simulink model "verify_clq2pressuredropcoeff_mdl"  (R2016b)
settings: Solver=VariableStepDiscrete  StartTime=0.0  StopTime=10.0  MaxStep=0.1  RelTol=1e-3  EnableMultiTasking=on
libraries: carnot x3, simulink x1
settings Model: Creator=drhf  LastModifiedBy=drhf
settings DataIOCC: LimitDataPoints=on  SaveFormat=Array
settings OptimizationCC: ExpressionDepthLimit=2147483647  LifeSpan=inf
settings DebuggingCC: UnderspecifiedInitializationDetection=Classic  MergeDetectMultiDrivingBlocksExec=none  SolverPrmCheckMsg=warning  StateNameClashWarn=warning  SFUnexpectedBacktrackingDiag=warning  SFNoUnconditionalDefaultTransitionDiag=warning  SFExecutionAtInitializationDiag=none
settings HardwareCC: ProdBitPerPointer=32  ProdBitPerSizeT=32  ProdBitPerPtrDiffT=32  ProdLargestAtomicFloat=None  ProdIntDivRoundTo=Undefined  ProdEndianess=Unspecified  ProdWordSize=32  ProdHWDeviceType=32-bit Generic
settings ModelReferenceCC: PropagateSignalLabelsOutOfModel=off
settings GRTTargetCC: TargetLangStandard=C89/C90 (ANSI)  GeneratePreprocessorConditionals=Disable all  CombineOutputUpdateFcns=off  GRTInterface=on
settings ConfigComp: CovMetricSettings=dw  CovHtmlReporting=on  CovSaveCumulativeToWorkspaceVar=on  CovSaveSingleToWorkspaceVar=on  CovExternalEMLEnable=off

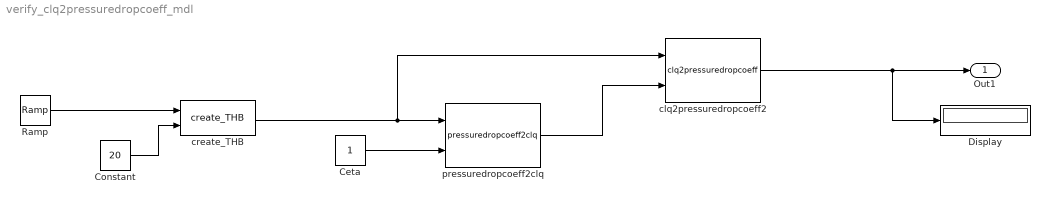
== system verify_clq2pressuredropcoeff_mdl ==
  Ceta : Constant
  Constant : Constant  Value=20
  Display : Display
  Ramp : simulink/Sources/Ramp  slope=0.01  start=0  X0=0
  clq2pressuredropcoeff2 : carnot/Basic/Pressure_Drop/clq2pressuredropcoeff
  create_THB : carnot/Source/Simple/create_THB  p=1e5  fluid=Water  mix=0  mix2=0  mix3=0  dia=0.02  hgt=0  mID=Pressure Drop from Massflow
  pressuredropcoeff2clq : carnot/Basic/Pressure_Drop/pressuredropcoeff2clq
  Out1 : Outport  SampleTime=1
  wires:
  clq2pressuredropcoeff2/1 -> Display/1, Out1/1
  Ramp/1 -> create_THB/1
  Constant/1 -> create_THB/2
  create_THB/1 -> clq2pressuredropcoeff2/1, pressuredropcoeff2clq/1
  Ceta/1 -> pressuredropcoeff2clq/2
  pressuredropcoeff2clq/1 -> clq2pressuredropcoeff2/2
